simulink library "reaction_wheel_assembly_lib"  (R2018b)
settings: Solver=VariableStepAuto  StartTime=0.0  StopTime=10.0  RelTol=1e-3
undefined symbols (not defined in the file): simParams
libraries: rpm_2_torque_lib x4, reaction_wheel_PID_lib x4, rw_motor_lib_disc x4, rwa_power_lib x1
settings Model: Creator=unsik  LastModifiedBy=Taylor
settings SFSimCC: SimUseLocalCustomCode=off
settings RTWCC: RTWUseLocalCustomCode=off
settings CodeAppCC: StateflowObjectComments=on

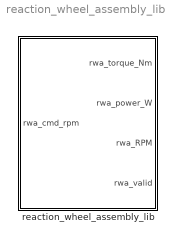
== system reaction_wheel_assembly_lib ==
  reaction_wheel_assembly_lib : Subsystem

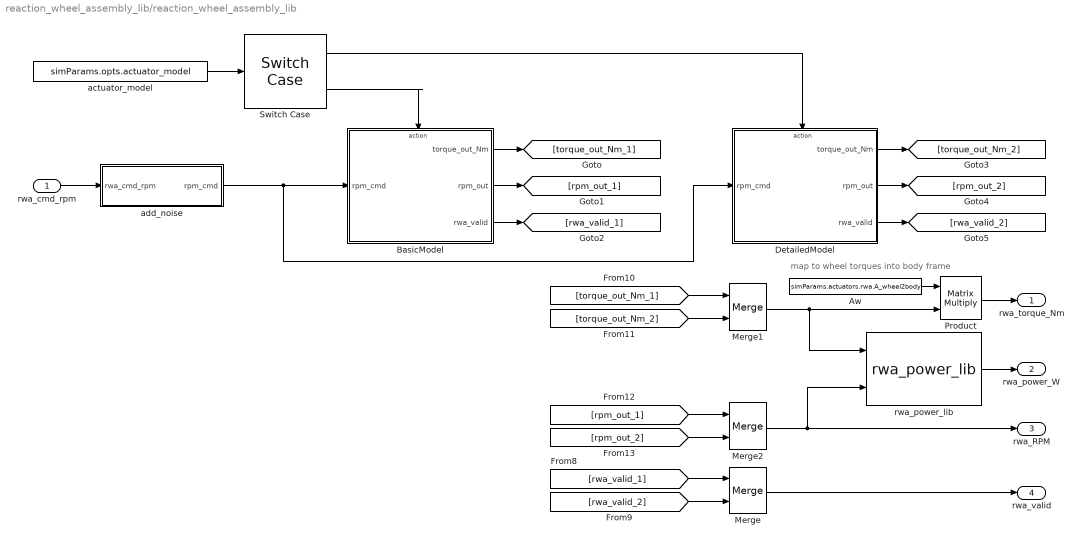
== system reaction_wheel_assembly_lib/reaction_wheel_assembly_lib ==
  note: map to wheel torques into body frame
  rwa_cmd_rpm : Inport
  Aw : Constant  Value=simParams.actuators.rwa.A_wheel2body  SampleTime=simParams.sample_time_s
  BasicModel : Subsystem  TreatAsAtomicUnit=on
  DetailedModel : Subsystem  TreatAsAtomicUnit=on
  Merge : Merge
  Merge1 : Merge
  Merge2 : Merge
  Product : Product  Multiplication=Matrix(*)
  Switch Case : SwitchCase
  actuator_model : Constant  Value=simParams.opts.actuator_model
  add_noise : Subsystem
  rwa_power_lib : rwa_power_lib/rwa_power_lib  SystemSampleTime=-1
  rwa_torque_Nm : Outport
  rwa_power_W : Outport  Port=2
  rwa_RPM : Outport  Port=3
  rwa_valid : Outport  Port=4
  wires:
  Product/1 -> rwa_torque_Nm/1
  Merge1/1 -> Product/2, rwa_power_lib/1
  Aw/1 -> Product/1
  rwa_power_lib/1 -> rwa_power_W/1
  Merge2/1 -> rwa_RPM/1, rwa_power_lib/2
  rwa_cmd_rpm/1 -> add_noise/1(rwa_cmd_rpm)
  actuator_model/1 -> Switch Case/1
  Switch Case/2 -> BasicModel/Action
  Switch Case/1 -> DetailedModel/Action
  add_noise/1(rpm_cmd) -> DetailedModel/1(rpm_cmd), BasicModel/1(rpm_cmd)
  BasicModel/1(torque_out_Nm) -> [torque_out_Nm_1]
  BasicModel/2(rpm_out) -> [rpm_out_1]
  BasicModel/3(rwa_valid) -> [rwa_valid_1]
  DetailedModel/3(rwa_valid) -> [rwa_valid_2]
  DetailedModel/2(rpm_out) -> [rpm_out_2]
  DetailedModel/1(torque_out_Nm) -> [torque_out_Nm_2]
  Merge/1 -> rwa_valid/1
  [rwa_valid_1] -> Merge/1
  [rwa_valid_2] -> Merge/2
  [torque_out_Nm_2] -> Merge1/2
  [torque_out_Nm_1] -> Merge1/1
  [rpm_out_1] -> Merge2/1
  [rpm_out_2] -> Merge2/2

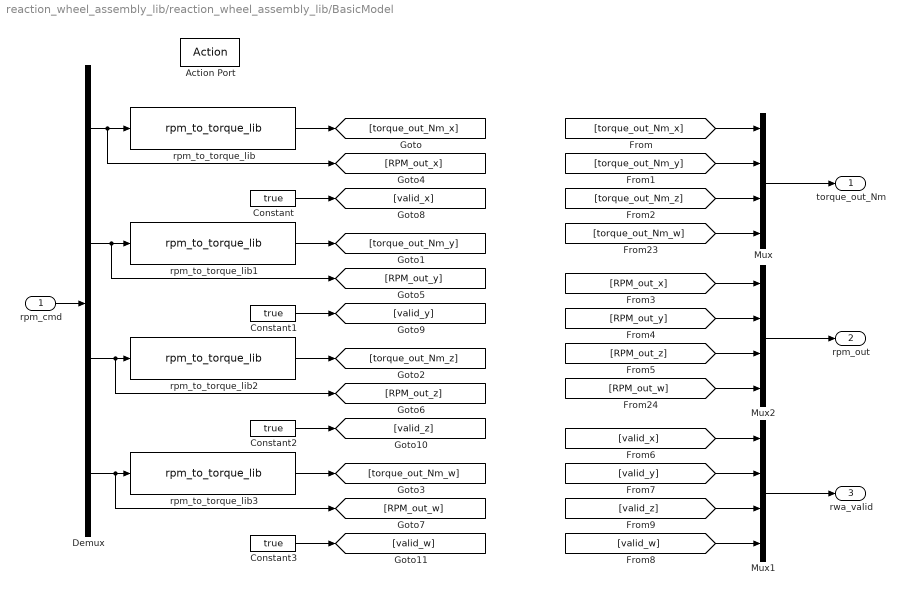
== system reaction_wheel_assembly_lib/reaction_wheel_assembly_lib/BasicModel ==
  rpm_cmd : Inport
  Action Port : ActionPort  ActionType=default
  Constant{,1..3} (4 alike) : Constant  Value=true
  Demux : Demux  Outputs=[1 1 1 1]
  Mux : Mux  Inputs=[1;1;1;1]
  Mux1 : Mux  Inputs=[1;1;1;1]
  Mux2 : Mux  Inputs=[1;1;1;1]
  rpm_to_torque_lib{,1..3} (4 alike) : rpm_2_torque_lib/rpm_to_torque_lib  SystemSampleTime=-1
  torque_out_Nm : Outport
  rpm_out : Outport  Port=2
  rwa_valid : Outport  Port=3
  wires:
  rpm_to_torque_lib/1 -> [torque_out_Nm_x]
  Constant/1 -> [valid_x]
  Demux/3 -> [RPM_out_z], rpm_to_torque_lib2/1
  Demux/4 -> [RPM_out_w], rpm_to_torque_lib3/1
  Demux/2 -> [RPM_out_y], rpm_to_torque_lib1/1
  rpm_to_torque_lib1/1 -> [torque_out_Nm_y]
  Constant3/1 -> [valid_w]
  Constant2/1 -> [valid_z]
  Constant1/1 -> [valid_y]
  rpm_to_torque_lib3/1 -> [torque_out_Nm_w]
  rpm_to_torque_lib2/1 -> [torque_out_Nm_z]
  [torque_out_Nm_z] -> Mux/3
  [torque_out_Nm_w] -> Mux/4
  [torque_out_Nm_x] -> Mux/1
  [torque_out_Nm_y] -> Mux/2
  [RPM_out_w] -> Mux2/4
  [RPM_out_z] -> Mux2/3
  [RPM_out_y] -> Mux2/2
  [RPM_out_x] -> Mux2/1
  Mux/1 -> torque_out_Nm/1
  Mux2/1 -> rpm_out/1
  [valid_x] -> Mux1/1
  [valid_y] -> Mux1/2
  [valid_z] -> Mux1/3
  [valid_w] -> Mux1/4
  Mux1/1 -> rwa_valid/1
  Demux/1 -> [RPM_out_x], rpm_to_torque_lib/1
  rpm_cmd/1 -> Demux/1

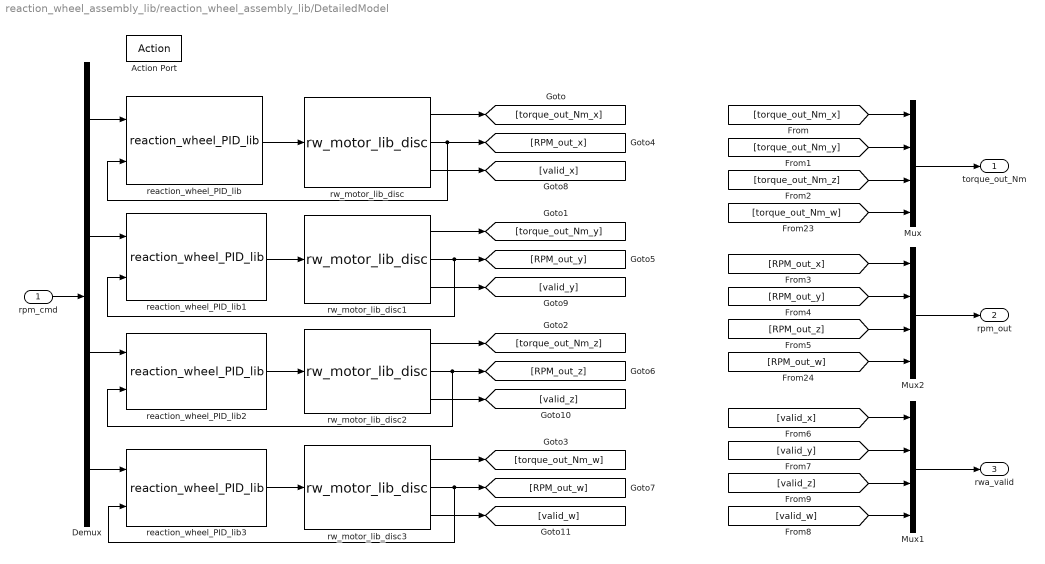
== system reaction_wheel_assembly_lib/reaction_wheel_assembly_lib/DetailedModel ==
  rpm_cmd : Inport
  Action Port : ActionPort  ActionType=case
  Demux : Demux  Outputs=[1 1 1 1]
  Mux : Mux  Inputs=[1;1;1;1]
  Mux1 : Mux  Inputs=[1;1;1;1]
  Mux2 : Mux  Inputs=[1;1;1;1]
  reaction_wheel_PID_lib{,1..3} (4 alike) : reaction_wheel_PID_lib/reaction_wheel_PID_lib  SystemSampleTime=-1
  rw_motor_lib_disc : rw_motor_lib_disc/rw_motor_lib_disc  id_a=1
  rw_motor_lib_disc1 : rw_motor_lib_disc/rw_motor_lib_disc  id_a=2
  rw_motor_lib_disc2 : rw_motor_lib_disc/rw_motor_lib_disc  id_a=3
  rw_motor_lib_disc3 : rw_motor_lib_disc/rw_motor_lib_disc  id_a=4
  torque_out_Nm : Outport
  rpm_out : Outport  Port=2
  rwa_valid : Outport  Port=3
  wires:
  rw_motor_lib_disc2/2 -> [RPM_out_z], reaction_wheel_PID_lib2/2
  rw_motor_lib_disc1/3 -> [valid_y]
  rw_motor_lib_disc1/2 -> [RPM_out_y], reaction_wheel_PID_lib1/2
  rw_motor_lib_disc2/3 -> [valid_z]
  Demux/3 -> reaction_wheel_PID_lib2/1
  rw_motor_lib_disc2/1 -> [torque_out_Nm_z]
  rw_motor_lib_disc3/2 -> [RPM_out_w], reaction_wheel_PID_lib3/2
  rw_motor_lib_disc/3 -> [valid_x]
  reaction_wheel_PID_lib/1 -> rw_motor_lib_disc/1
  rw_motor_lib_disc3/3 -> [valid_w]
  Demux/2 -> reaction_wheel_PID_lib1/1
  reaction_wheel_PID_lib2/1 -> rw_motor_lib_disc2/1
  rw_motor_lib_disc/1 -> [torque_out_Nm_x]
  Demux/4 -> reaction_wheel_PID_lib3/1
  rw_motor_lib_disc1/1 -> [torque_out_Nm_y]
  rw_motor_lib_disc/2 -> [RPM_out_x], reaction_wheel_PID_lib/2
  rw_motor_lib_disc3/1 -> [torque_out_Nm_w]
  reaction_wheel_PID_lib1/1 -> rw_motor_lib_disc1/1
  reaction_wheel_PID_lib3/1 -> rw_motor_lib_disc3/1
  Mux1/1 -> rwa_valid/1
  Mux2/1 -> rpm_out/1
  [torque_out_Nm_x] -> Mux/1
  Mux/1 -> torque_out_Nm/1
  [valid_z] -> Mux1/3
  [valid_y] -> Mux1/2
  [valid_w] -> Mux1/4
  [valid_x] -> Mux1/1
  [torque_out_Nm_w] -> Mux/4
  [torque_out_Nm_y] -> Mux/2
  [RPM_out_y] -> Mux2/2
  [RPM_out_w] -> Mux2/4
  [RPM_out_x] -> Mux2/1
  [RPM_out_z] -> Mux2/3
  [torque_out_Nm_z] -> Mux/3
  Demux/1 -> reaction_wheel_PID_lib/1
  rpm_cmd/1 -> Demux/1

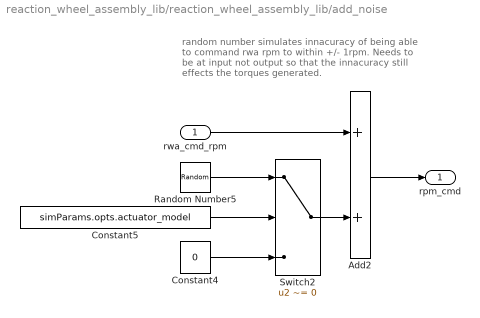
== system reaction_wheel_assembly_lib/reaction_wheel_assembly_lib/add_noise ==
  note: random number simulates innacuracy of being able to command rwa rpm to within +/- 1rpm. Needs to be at input not output so that the innacuracy still effects the torques generated.
  rwa_cmd_rpm : Inport
  Add2 : Sum
  Constant4 : Constant  Value=0
  Constant5 : Constant  Value=simParams.opts.actuator_model
  Random Number5 : RandomNumber  Variance=simParams.actuators.rwa.rpm_variance  Seed=simParams.actuators.rwa.seed  SampleTime=simParams.sample_time_s
  Switch2 : Switch  Criteria=u2 ~= 0
  rpm_cmd : Outport
  wires:
  Constant4/1 -> Switch2/3
  Switch2/1 -> Add2/2
  Constant5/1 -> Switch2/2
  Random Number5/1 -> Switch2/1
  rwa_cmd_rpm/1 -> Add2/1
  Add2/1 -> rpm_cmd/1
